simulink model "ieee30"  (R2017a)
settings: Solver=VariableStepDiscrete  StartTime=0.0  StopTime=0.012  MaxStep=1e-4  RelTol=1e-3
undefined symbols (not defined in the file): Angle, Magnitude
libraries: powerlib x548
(part 3 of 4)

== system ieee30/Bus29 ==
  I2927 : powerlib/Measurements/Three-Phase V-I Measurement  VoltageMeasurement=no  SetLabelV=off  LabelV=Vabc  Vpu=off  VpuLL=off  CurrentMeasurement=yes  SetLabelI=on  LabelI=I2927  Ipu=off  Pbase=100e6  Vbase=500e3  OutputType=Magnitude-Angle  PhasorSimulation=on  PSBequivalent=0
  Load29 : powerlib/Measurements/Three-Phase V-I Measurement  VoltageMeasurement=no  SetLabelV=off  LabelV=V21  Vpu=off  VpuLL=off  CurrentMeasurement=no  SetLabelI=off  LabelI=I2224  Ipu=off  Pbase=100e6  Vbase=500e3  OutputType=Complex  PhasorSimulation=on  PSBequivalent=0
  To Workspace1 : ToWorkspace  VariableName=V29  SaveFormat=Timeseries  SampleTime=0.01
  To Workspace2 : ToWorkspace  VariableName=I2927  SaveFormat=Timeseries  SampleTime=0.01
  To Workspace3 : ToWorkspace  VariableName=I2930  SaveFormat=Timeseries  SampleTime=0.01
  V29 I2930 : powerlib/Measurements/Three-Phase V-I Measurement  VoltageMeasurement=phase-to-phase  SetLabelV=on  LabelV=V29  Vpu=off  VpuLL=off  CurrentMeasurement=yes  SetLabelI=on  LabelI=I2930  Ipu=off  Pbase=100e6  Vbase=500e3  OutputType=Magnitude-Angle  PhasorSimulation=on  PSBequivalent=0
  I2930A : PMIOPort  Port=1  Side=Right
  I2930B : PMIOPort  Port=2  Side=Right
  I2930C : PMIOPort  Port=3  Side=Right
  I2927A : PMIOPort  Port=4  Side=Right
  I2927B : PMIOPort  Port=5  Side=Right
  I2927C : PMIOPort  Port=6  Side=Right
  Load29A : PMIOPort  Port=7  Side=Left
  Load29B : PMIOPort  Port=8  Side=Left
  Load29C : PMIOPort  Port=9  Side=Left
  wires:
  [V29] -> To Workspace1/1
  [I2927] -> To Workspace2/1
  [I2930] -> To Workspace3/1
  connections:
  V29 I2930/RConn2 -- I2930B/RConn1
  I2927/RConn1 -- I2927A/RConn1
  V29 I2930/RConn1 -- I2930A/RConn1
  I2927/RConn2 -- I2927B/RConn1
  I2927/RConn3 -- I2927C/RConn1
  V29 I2930/RConn3 -- I2930C/RConn1
  V29 I2930/LConn1 -- Load29/LConn1 -- I2927/LConn1
  V29 I2930/LConn2 -- Load29/LConn2 -- I2927/LConn2
  V29 I2930/LConn3 -- Load29/LConn3 -- I2927/LConn3
  Load29/RConn1 -- Load29A/RConn1
  Load29/RConn2 -- Load29B/RConn1
  Load29/RConn3 -- Load29C/RConn1

== system ieee30/Bus3 ==
  I34 : powerlib/Measurements/Three-Phase V-I Measurement  VoltageMeasurement=no  SetLabelV=off  LabelV=V3  Vpu=off  VpuLL=off  CurrentMeasurement=yes  SetLabelI=on  LabelI=I34  Ipu=off  Pbase=100e6  Vbase=500e3  OutputType=Magnitude-Angle  PhasorSimulation=on  PSBequivalent=0
  Load3 : powerlib/Measurements/Three-Phase V-I Measurement  VoltageMeasurement=no  SetLabelV=off  LabelV=V3  Vpu=off  VpuLL=off  CurrentMeasurement=no  SetLabelI=off  LabelI=I31  Ipu=off  Pbase=100e6  Vbase=500e3  OutputType=Complex  PhasorSimulation=on  PSBequivalent=0
  To Workspace1 : ToWorkspace  VariableName=I34  SaveFormat=Timeseries  SampleTime=0.01
  To Workspace2 : ToWorkspace  VariableName=I31  SaveFormat=Timeseries  SampleTime=0.01
  To Workspace3 : ToWorkspace  VariableName=V3  SaveFormat=Timeseries  SampleTime=0.01
  V3 I31 : powerlib/Measurements/Three-Phase V-I Measurement  VoltageMeasurement=phase-to-phase  SetLabelV=on  LabelV=V3  Vpu=off  VpuLL=off  CurrentMeasurement=yes  SetLabelI=on  LabelI=I31  Ipu=off  Pbase=100e6  Vbase=500e3  OutputType=Magnitude-Angle  PhasorSimulation=on  PSBequivalent=0
  I31A : PMIOPort  Port=1  Side=Left
  I31B : PMIOPort  Port=2  Side=Left
  I31C : PMIOPort  Port=3  Side=Left
  Load3A : PMIOPort  Port=4  Side=Left
  Load3B : PMIOPort  Port=5  Side=Left
  Load3C : PMIOPort  Port=6  Side=Left
  I34A : PMIOPort  Port=7  Side=Right
  I34B : PMIOPort  Port=8  Side=Right
  I34C : PMIOPort  Port=9  Side=Right
  wires:
  [I31] -> To Workspace2/1
  [V3] -> To Workspace3/1
  [I34] -> To Workspace1/1
  connections:
  I31A/RConn1 -- V3 I31/RConn1
  I31B/RConn1 -- V3 I31/RConn2
  I31C/RConn1 -- V3 I31/RConn3
  Load3/RConn3 -- Load3C/RConn1
  Load3/RConn1 -- Load3A/RConn1
  Load3/RConn2 -- Load3B/RConn1
  I34/RConn3 -- I34C/RConn1
  I34/RConn1 -- I34A/RConn1
  I34/RConn2 -- I34B/RConn1
  V3 I31/LConn1 -- I34/LConn1 -- Load3/LConn1
  V3 I31/LConn2 -- Load3/LConn2 -- I34/LConn2
  V3 I31/LConn3 -- Load3/LConn3 -- I34/LConn3

== system ieee30/Bus30 ==
  I3029 : powerlib/Measurements/Three-Phase V-I Measurement  VoltageMeasurement=no  SetLabelV=off  LabelV=Vabc  Vpu=off  VpuLL=off  CurrentMeasurement=yes  SetLabelI=on  LabelI=I3029  Ipu=off  Pbase=100e6  Vbase=500e3  OutputType=Magnitude-Angle  PhasorSimulation=on  PSBequivalent=0
  Load30 : powerlib/Measurements/Three-Phase V-I Measurement  VoltageMeasurement=no  SetLabelV=off  LabelV=V21  Vpu=off  VpuLL=off  CurrentMeasurement=no  SetLabelI=off  LabelI=I2224  Ipu=off  Pbase=100e6  Vbase=500e3  OutputType=Complex  PhasorSimulation=on  PSBequivalent=0
  To Workspace1 : ToWorkspace  VariableName=V30  SaveFormat=Timeseries  SampleTime=0.01
  To Workspace2 : ToWorkspace  VariableName=I3027  SaveFormat=Timeseries  SampleTime=0.01
  To Workspace3 : ToWorkspace  VariableName=I3029  SaveFormat=Timeseries  SampleTime=0.01
  V30 I3027 : powerlib/Measurements/Three-Phase V-I Measurement  VoltageMeasurement=phase-to-phase  SetLabelV=on  LabelV=V30  Vpu=off  VpuLL=off  CurrentMeasurement=yes  SetLabelI=on  LabelI=I3027  Ipu=off  Pbase=100e6  Vbase=500e3  OutputType=Magnitude-Angle  PhasorSimulation=on  PSBequivalent=0
  I3029A : PMIOPort  Port=1  Side=Right
  I3029B : PMIOPort  Port=2  Side=Right
  I3029C : PMIOPort  Port=3  Side=Right
  I3027A : PMIOPort  Port=4  Side=Right
  I3027B : PMIOPort  Port=5  Side=Right
  I3027C : PMIOPort  Port=6  Side=Right
  Load30A : PMIOPort  Port=7  Side=Left
  Load30B : PMIOPort  Port=8  Side=Left
  Load30C : PMIOPort  Port=9  Side=Left
  wires:
  [V30] -> To Workspace1/1
  [I3027] -> To Workspace2/1
  [I3029] -> To Workspace3/1
  connections:
  V30 I3027/RConn2 -- I3027B/RConn1
  I3029/RConn1 -- I3029A/RConn1
  V30 I3027/RConn1 -- I3027A/RConn1
  I3029/RConn2 -- I3029B/RConn1
  I3029/RConn3 -- I3029C/RConn1
  V30 I3027/RConn3 -- I3027C/RConn1
  V30 I3027/LConn1 -- Load30/LConn1 -- I3029/LConn1
  V30 I3027/LConn2 -- Load30/LConn2 -- I3029/LConn2
  V30 I3027/LConn3 -- Load30/LConn3 -- I3029/LConn3
  Load30/RConn1 -- Load30A/RConn1
  Load30/RConn2 -- Load30B/RConn1
  Load30/RConn3 -- Load30C/RConn1

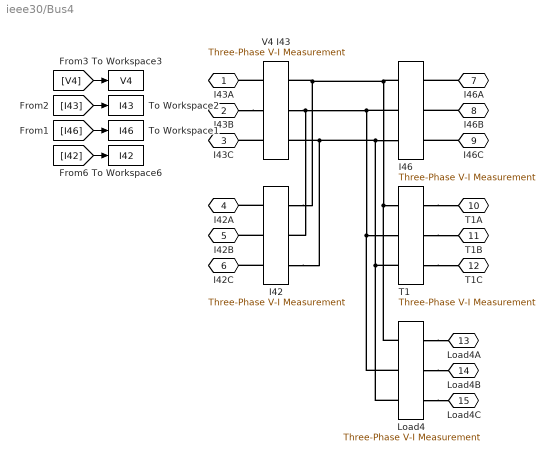
== system ieee30/Bus4 ==
  I42 : powerlib/Measurements/Three-Phase V-I Measurement  VoltageMeasurement=no  SetLabelV=off  LabelV=V4  Vpu=off  VpuLL=off  CurrentMeasurement=yes  SetLabelI=on  LabelI=I42  Ipu=off  Pbase=100e6  Vbase=500e3  OutputType=Magnitude-Angle  PhasorSimulation=on  PSBequivalent=0
  I46 : powerlib/Measurements/Three-Phase V-I Measurement  VoltageMeasurement=no  SetLabelV=off  LabelV=V4  Vpu=off  VpuLL=off  CurrentMeasurement=yes  SetLabelI=on  LabelI=I46  Ipu=off  Pbase=100e6  Vbase=500e3  OutputType=Magnitude-Angle  PhasorSimulation=on  PSBequivalent=0
  Load4 : powerlib/Measurements/Three-Phase V-I Measurement  VoltageMeasurement=no  SetLabelV=off  LabelV=V4  Vpu=off  VpuLL=off  CurrentMeasurement=no  SetLabelI=off  LabelI=I412  Ipu=off  Pbase=100e6  Vbase=500e3  OutputType=Complex  PhasorSimulation=on  PSBequivalent=0
  T1 : powerlib/Measurements/Three-Phase V-I Measurement  VoltageMeasurement=no  SetLabelV=off  LabelV=V4  Vpu=off  VpuLL=off  CurrentMeasurement=no  SetLabelI=off  LabelI=I412  Ipu=off  Pbase=100e6  Vbase=500e3  OutputType=Complex  PhasorSimulation=on  PSBequivalent=0
  To Workspace1 : ToWorkspace  VariableName=I46  SaveFormat=Timeseries  SampleTime=0.01
  To Workspace2 : ToWorkspace  VariableName=I43  SaveFormat=Timeseries  SampleTime=0.01
  To Workspace3 : ToWorkspace  VariableName=V4  SaveFormat=Timeseries  SampleTime=0.01
  To Workspace6 : ToWorkspace  VariableName=I42  SaveFormat=Timeseries  SampleTime=0.01
  V4 I43 : powerlib/Measurements/Three-Phase V-I Measurement  VoltageMeasurement=phase-to-phase  SetLabelV=on  LabelV=V4  Vpu=off  VpuLL=off  CurrentMeasurement=yes  SetLabelI=on  LabelI=I43  Ipu=off  Pbase=100e6  Vbase=500e3  OutputType=Magnitude-Angle  PhasorSimulation=on  PSBequivalent=0
  I43A : PMIOPort  Port=1  Side=Left
  I43B : PMIOPort  Port=2  Side=Left
  I43C : PMIOPort  Port=3  Side=Left
  I42A : PMIOPort  Port=4  Side=Left
  I42B : PMIOPort  Port=5  Side=Left
  I42C : PMIOPort  Port=6  Side=Left
  I46A : PMIOPort  Port=7  Side=Left
  I46B : PMIOPort  Port=8  Side=Left
  I46C : PMIOPort  Port=9  Side=Left
  T1A : PMIOPort  Port=10  Side=Right
  T1B : PMIOPort  Port=11  Side=Right
  T1C : PMIOPort  Port=12  Side=Right
  Load4A : PMIOPort  Port=13  Side=Right
  Load4B : PMIOPort  Port=14  Side=Right
  Load4C : PMIOPort  Port=15  Side=Right
  wires:
  [I46] -> To Workspace1/1
  [V4] -> To Workspace3/1
  [I43] -> To Workspace2/1
  [I42] -> To Workspace6/1
  connections:
  I43B/RConn1 -- V4 I43/RConn2
  V4 I43/RConn1 -- I43A/RConn1
  V4 I43/RConn3 -- I43C/RConn1
  T1/LConn3 -- V4 I43/LConn3 -- I42/LConn3 -- I46/LConn3 -- Load4/LConn3
  I46/LConn1 -- Load4/LConn1 -- T1/LConn1 -- I42/LConn1 -- V4 I43/LConn1
  V4 I43/LConn2 -- I46/LConn2 -- Load4/LConn2 -- T1/LConn2 -- I42/LConn2
  I42/RConn1 -- I42A/RConn1
  I42/RConn2 -- I42B/RConn1
  I42/RConn3 -- I42C/RConn1
  I46A/RConn1 -- I46/RConn1
  I46B/RConn1 -- I46/RConn2
  I46C/RConn1 -- I46/RConn3
  T1/RConn1 -- T1A/RConn1
  T1/RConn3 -- T1C/RConn1
  T1/RConn2 -- T1B/RConn1
  Load4/RConn1 -- Load4A/RConn1
  Load4/RConn2 -- Load4B/RConn1
  Load4/RConn3 -- Load4C/RConn1

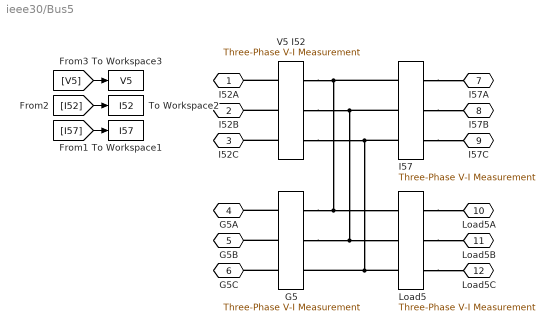
== system ieee30/Bus5 ==
  G5 : powerlib/Measurements/Three-Phase V-I Measurement  VoltageMeasurement=no  SetLabelV=off  LabelV=V5  Vpu=off  VpuLL=off  CurrentMeasurement=no  SetLabelI=off  LabelI=I52  Ipu=off  Pbase=100e6  Vbase=500e3  OutputType=Complex  PhasorSimulation=on  PSBequivalent=0
  I57 : powerlib/Measurements/Three-Phase V-I Measurement  VoltageMeasurement=no  SetLabelV=off  LabelV=V5  Vpu=off  VpuLL=off  CurrentMeasurement=yes  SetLabelI=on  LabelI=I57  Ipu=off  Pbase=100e6  Vbase=500e3  OutputType=Magnitude-Angle  PhasorSimulation=on  PSBequivalent=0
  Load5 : powerlib/Measurements/Three-Phase V-I Measurement  VoltageMeasurement=no  SetLabelV=off  LabelV=V5  Vpu=off  VpuLL=off  CurrentMeasurement=no  SetLabelI=off  LabelI=I52  Ipu=off  Pbase=100e6  Vbase=500e3  OutputType=Complex  PhasorSimulation=on  PSBequivalent=0
  To Workspace1 : ToWorkspace  VariableName=I57  SaveFormat=Timeseries  SampleTime=0.01
  To Workspace2 : ToWorkspace  VariableName=I52  SaveFormat=Timeseries  SampleTime=0.01
  To Workspace3 : ToWorkspace  VariableName=V5  SaveFormat=Timeseries  SampleTime=0.01
  V5 I52 : powerlib/Measurements/Three-Phase V-I Measurement  VoltageMeasurement=phase-to-phase  SetLabelV=on  LabelV=V5  Vpu=off  VpuLL=off  CurrentMeasurement=yes  SetLabelI=on  LabelI=I52  Ipu=off  Pbase=100e6  Vbase=500e3  OutputType=Magnitude-Angle  PhasorSimulation=on  PSBequivalent=0
  I52A : PMIOPort  Port=1  Side=Left
  I52B : PMIOPort  Port=2  Side=Left
  I52C : PMIOPort  Port=3  Side=Left
  G5A : PMIOPort  Port=4  Side=Right
  G5B : PMIOPort  Port=5  Side=Right
  G5C : PMIOPort  Port=6  Side=Right
  I57A : PMIOPort  Port=7  Side=Left
  I57B : PMIOPort  Port=8  Side=Left
  I57C : PMIOPort  Port=9  Side=Left
  Load5A : PMIOPort  Port=10  Side=Right
  Load5B : PMIOPort  Port=11  Side=Right
  Load5C : PMIOPort  Port=12  Side=Right
  wires:
  [I57] -> To Workspace1/1
  [V5] -> To Workspace3/1
  [I52] -> To Workspace2/1
  connections:
  V5 I52/RConn3 -- I52C/RConn1
  V5 I52/RConn2 -- I52B/RConn1
  V5 I52/RConn1 -- I52A/RConn1
  V5 I52/LConn1 -- I57/LConn1 -- Load5/LConn1 -- G5/LConn1
  V5 I52/LConn2 -- I57/LConn2 -- Load5/LConn2 -- G5/LConn2
  V5 I52/LConn3 -- I57/LConn3 -- G5/LConn3 -- Load5/LConn3
  G5/RConn1 -- G5A/RConn1
  G5/RConn3 -- G5C/RConn1
  G5/RConn2 -- G5B/RConn1
  I57/RConn3 -- I57C/RConn1
  I57/RConn1 -- I57A/RConn1
  I57/RConn2 -- I57B/RConn1
  Load5/RConn1 -- Load5A/RConn1
  Load5/RConn2 -- Load5B/RConn1
  Load5/RConn3 -- Load5C/RConn1

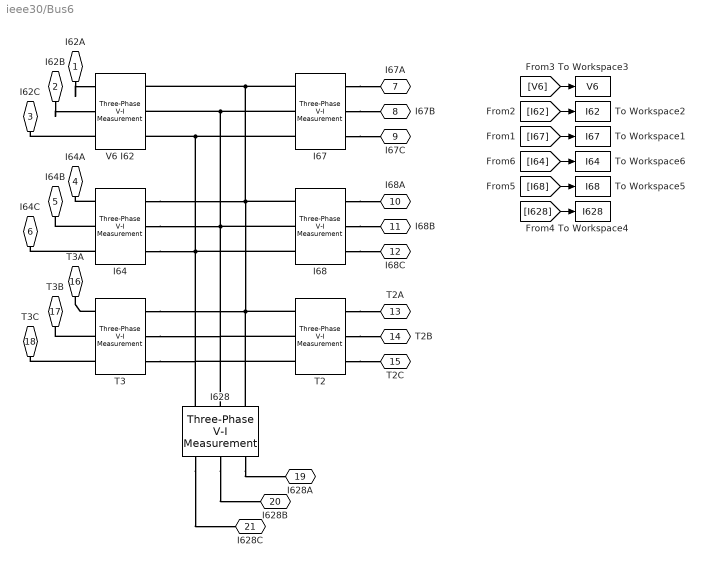
== system ieee30/Bus6 ==
  I628 : powerlib/Measurements/Three-Phase V-I Measurement  VoltageMeasurement=no  SetLabelV=off  LabelV=Vabc  Vpu=off  VpuLL=off  CurrentMeasurement=yes  SetLabelI=on  LabelI=I628  Ipu=off  Pbase=100e6  Vbase=500e3  OutputType=Magnitude-Angle  PhasorSimulation=on  PSBequivalent=0
  I64 : powerlib/Measurements/Three-Phase V-I Measurement  VoltageMeasurement=no  SetLabelV=off  LabelV=V6  Vpu=off  VpuLL=off  CurrentMeasurement=yes  SetLabelI=on  LabelI=I64  Ipu=off  Pbase=100e6  Vbase=500e3  OutputType=Magnitude-Angle  PhasorSimulation=on  PSBequivalent=0
  I67 : powerlib/Measurements/Three-Phase V-I Measurement  VoltageMeasurement=no  SetLabelV=off  LabelV=Vabc  Vpu=off  VpuLL=off  CurrentMeasurement=yes  SetLabelI=on  LabelI=I67  Ipu=off  Pbase=100e6  Vbase=500e3  OutputType=Magnitude-Angle  PhasorSimulation=on  PSBequivalent=0
  I68 : powerlib/Measurements/Three-Phase V-I Measurement  VoltageMeasurement=no  SetLabelV=off  LabelV=Vabc  Vpu=off  VpuLL=off  CurrentMeasurement=yes  SetLabelI=on  LabelI=I68  Ipu=off  Pbase=100e6  Vbase=500e3  OutputType=Magnitude-Angle  PhasorSimulation=on  PSBequivalent=0
  T2 : powerlib/Measurements/Three-Phase V-I Measurement  VoltageMeasurement=no  SetLabelV=off  LabelV=Vabc  Vpu=off  VpuLL=off  CurrentMeasurement=no  SetLabelI=off  LabelI=I69  Ipu=off  Pbase=100e6  Vbase=500e3  OutputType=Complex  PhasorSimulation=on  PSBequivalent=0
  T3 : powerlib/Measurements/Three-Phase V-I Measurement  VoltageMeasurement=no  SetLabelV=off  LabelV=Vabc  Vpu=off  VpuLL=off  CurrentMeasurement=no  SetLabelI=off  LabelI=I69  Ipu=off  Pbase=100e6  Vbase=500e3  OutputType=Complex  PhasorSimulation=on  PSBequivalent=0
  To Workspace1 : ToWorkspace  VariableName=I67  SaveFormat=Timeseries  SampleTime=0.01
  To Workspace2 : ToWorkspace  VariableName=I62  SaveFormat=Timeseries  SampleTime=0.01
  To Workspace3 : ToWorkspace  VariableName=V6  SaveFormat=Timeseries  SampleTime=0.01
  To Workspace4 : ToWorkspace  VariableName=I628  SaveFormat=Timeseries  SampleTime=0.01
  To Workspace5 : ToWorkspace  VariableName=I68  SaveFormat=Timeseries  SampleTime=0.01
  To Workspace6 : ToWorkspace  VariableName=I64  SaveFormat=Timeseries  SampleTime=0.01
  V6 I62 : powerlib/Measurements/Three-Phase V-I Measurement  VoltageMeasurement=phase-to-phase  SetLabelV=on  LabelV=V6  Vpu=off  VpuLL=off  CurrentMeasurement=yes  SetLabelI=on  LabelI=I62  Ipu=off  Pbase=100e6  Vbase=500e3  OutputType=Magnitude-Angle  PhasorSimulation=on  PSBequivalent=0
  I62A : PMIOPort  Port=1  Side=Left
  I62B : PMIOPort  Port=2  Side=Left
  I62C : PMIOPort  Port=3  Side=Left
  I64A : PMIOPort  Port=4  Side=Right
  I64B : PMIOPort  Port=5  Side=Right
  I64C : PMIOPort  Port=6  Side=Right
  I67A : PMIOPort  Port=7  Side=Left
  I67B : PMIOPort  Port=8  Side=Left
  I67C : PMIOPort  Port=9  Side=Left
  I68A : PMIOPort  Port=10  Side=Left
  I68B : PMIOPort  Port=11  Side=Left
  I68C : PMIOPort  Port=12  Side=Left
  T2A : PMIOPort  Port=13  Side=Right
  T2B : PMIOPort  Port=14  Side=Right
  T2C : PMIOPort  Port=15  Side=Right
  T3A : PMIOPort  Port=16  Side=Right
  T3B : PMIOPort  Port=17  Side=Right
  T3C : PMIOPort  Port=18  Side=Right
  I628A : PMIOPort  Port=19  Side=Right
  I628B : PMIOPort  Port=20  Side=Right
  I628C : PMIOPort  Port=21  Side=Right
  wires:
  [I67] -> To Workspace1/1
  [V6] -> To Workspace3/1
  [I62] -> To Workspace2/1
  [I628] -> To Workspace4/1
  [I64] -> To Workspace6/1
  [I68] -> To Workspace5/1
  connections:
  I62A/RConn1 -- V6 I62/RConn1
  I62B/RConn1 -- V6 I62/RConn2
  I64/LConn1 -- I68/LConn1 -- I67/LConn1 -- V6 I62/LConn1 -- I628/LConn3 -- T3/LConn1 -- T2/LConn1
  I64/LConn2 -- I68/LConn2 -- I67/LConn2 -- V6 I62/LConn2 -- I628/LConn2 -- T3/LConn2 -- T2/LConn2
  I64/LConn3 -- I68/LConn3 -- I67/LConn3 -- V6 I62/LConn3 -- I628/LConn1 -- T3/LConn3 -- T2/LConn3
  V6 I62/RConn3 -- I62C/RConn1
  I64/RConn3 -- I64C/RConn1
  I64/RConn2 -- I64B/RConn1
  I64/RConn1 -- I64A/RConn1
  I67/RConn1 -- I67A/RConn1
  I67/RConn3 -- I67C/RConn1
  I67/RConn2 -- I67B/RConn1
  I68/RConn3 -- I68C/RConn1
  I68/RConn1 -- I68A/RConn1
  I68/RConn2 -- I68B/RConn1
  T2/RConn2 -- T2B/RConn1
  T2/RConn3 -- T2C/RConn1
  T2/RConn1 -- T2A/RConn1
  T3/RConn3 -- T3C/RConn1
  T3/RConn1 -- T3A/RConn1
  T3/RConn2 -- T3B/RConn1
  I628/RConn1 -- I628C/RConn1
  I628/RConn3 -- I628A/RConn1
  I628/RConn2 -- I628B/RConn1

== system ieee30/Bus7 ==
  I76 : powerlib/Measurements/Three-Phase V-I Measurement  VoltageMeasurement=no  SetLabelV=off  LabelV=V7  Vpu=off  VpuLL=off  CurrentMeasurement=yes  SetLabelI=on  LabelI=I76  Ipu=off  Pbase=100e6  Vbase=500e3  OutputType=Magnitude-Angle  PhasorSimulation=on  PSBequivalent=0
  Load7 : powerlib/Measurements/Three-Phase V-I Measurement  VoltageMeasurement=no  SetLabelV=off  LabelV=V7  Vpu=off  VpuLL=off  CurrentMeasurement=no  SetLabelI=off  LabelI=I57  Ipu=off  Pbase=100e6  Vbase=500e3  OutputType=Complex  PhasorSimulation=on  PSBequivalent=0
  To Workspace1 : ToWorkspace  VariableName=I76  SaveFormat=Timeseries  SampleTime=0.01
  To Workspace2 : ToWorkspace  VariableName=I75  SaveFormat=Timeseries  SampleTime=0.01
  To Workspace3 : ToWorkspace  VariableName=V7  SaveFormat=Timeseries  SampleTime=0.01
  V7 I75 : powerlib/Measurements/Three-Phase V-I Measurement  VoltageMeasurement=phase-to-phase  SetLabelV=on  LabelV=V7  Vpu=off  VpuLL=off  CurrentMeasurement=yes  SetLabelI=on  LabelI=I75  Ipu=off  Pbase=100e6  Vbase=500e3  OutputType=Magnitude-Angle  PhasorSimulation=on  PSBequivalent=0
  Load7A : PMIOPort  Port=1  Side=Left
  Load7B : PMIOPort  Port=2  Side=Left
  Load7C : PMIOPort  Port=3  Side=Left
  I75A : PMIOPort  Port=4  Side=Left
  I75B : PMIOPort  Port=5  Side=Left
  I75C : PMIOPort  Port=6  Side=Left
  I76A : PMIOPort  Port=7  Side=Left
  I76B : PMIOPort  Port=8  Side=Left
  I76C : PMIOPort  Port=9  Side=Left
  wires:
  [I76] -> To Workspace1/1
  [V7] -> To Workspace3/1
  [I75] -> To Workspace2/1
  connections:
  I76/RConn3 -- I76C/RConn1
  V7 I75/RConn3 -- I75C/RConn1
  V7 I75/RConn2 -- I75B/RConn1
  V7 I75/RConn1 -- I75A/RConn1
  I76/RConn2 -- I76B/RConn1
  I76/RConn1 -- I76A/RConn1
  V7 I75/LConn1 -- Load7/LConn1 -- I76/LConn1
  V7 I75/LConn2 -- Load7/LConn2 -- I76/LConn2
  I76/LConn3 -- Load7/LConn3 -- V7 I75/LConn3
  Load7A/RConn1 -- Load7/RConn1
  Load7/RConn2 -- Load7B/RConn1
  Load7C/RConn1 -- Load7/RConn3

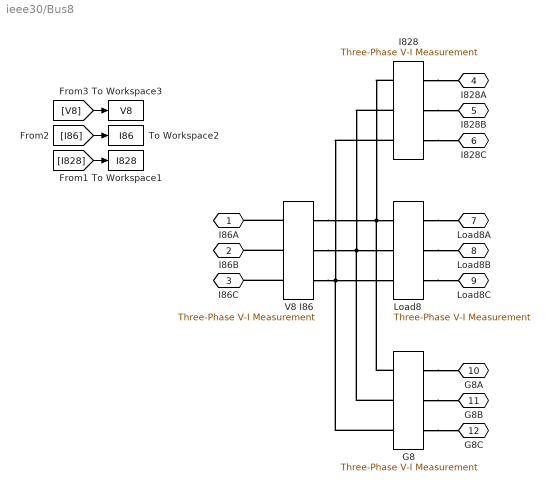
== system ieee30/Bus8 ==
  G8 : powerlib/Measurements/Three-Phase V-I Measurement  VoltageMeasurement=no  SetLabelV=off  LabelV=Vabc  Vpu=off  VpuLL=off  CurrentMeasurement=no  SetLabelI=off  LabelI=Iabc  Ipu=off  Pbase=100e6  Vbase=500e3  OutputType=Complex  PhasorSimulation=on  PSBequivalent=0
  I828 : powerlib/Measurements/Three-Phase V-I Measurement  VoltageMeasurement=no  SetLabelV=off  LabelV=V8  Vpu=off  VpuLL=off  CurrentMeasurement=yes  SetLabelI=on  LabelI=I828  Ipu=off  Pbase=100e6  Vbase=500e3  OutputType=Magnitude-Angle  PhasorSimulation=on  PSBequivalent=0
  Load8 : powerlib/Measurements/Three-Phase V-I Measurement  VoltageMeasurement=no  SetLabelV=off  LabelV=Vabc  Vpu=off  VpuLL=off  CurrentMeasurement=no  SetLabelI=off  LabelI=Iabc  Ipu=off  Pbase=100e6  Vbase=500e3  OutputType=Complex  PhasorSimulation=on  PSBequivalent=0
  To Workspace1 : ToWorkspace  VariableName=I828  SaveFormat=Timeseries  SampleTime=0.01
  To Workspace2 : ToWorkspace  VariableName=I86  SaveFormat=Timeseries  SampleTime=0.01
  To Workspace3 : ToWorkspace  VariableName=V8  SaveFormat=Timeseries  SampleTime=0.01
  V8 I86 : powerlib/Measurements/Three-Phase V-I Measurement  VoltageMeasurement=phase-to-phase  SetLabelV=on  LabelV=V8  Vpu=off  VpuLL=off  CurrentMeasurement=yes  SetLabelI=on  LabelI=I86  Ipu=off  Pbase=100e6  Vbase=500e3  OutputType=Magnitude-Angle  PhasorSimulation=on  PSBequivalent=0
  I86A : PMIOPort  Port=1  Side=Left
  I86B : PMIOPort  Port=2  Side=Left
  I86C : PMIOPort  Port=3  Side=Left
  I828A : PMIOPort  Port=4  Side=Right
  I828B : PMIOPort  Port=5  Side=Right
  I828C : PMIOPort  Port=6  Side=Right
  Load8A : PMIOPort  Port=7  Side=Right
  Load8B : PMIOPort  Port=8  Side=Right
  Load8C : PMIOPort  Port=9  Side=Right
  G8A : PMIOPort  Port=10  Side=Right
  G8B : PMIOPort  Port=11  Side=Right
  G8C : PMIOPort  Port=12  Side=Right
  wires:
  [I828] -> To Workspace1/1
  [V8] -> To Workspace3/1
  [I86] -> To Workspace2/1
  connections:
  V8 I86/RConn3 -- I86C/RConn1
  Load8/RConn3 -- Load8C/RConn1
  Load8/RConn2 -- Load8B/RConn1
  V8 I86/RConn2 -- I86B/RConn1
  Load8/RConn1 -- Load8A/RConn1
  V8 I86/RConn1 -- I86A/RConn1
  V8 I86/LConn1 -- I828/LConn1 -- G8/LConn1 -- Load8/LConn1
  V8 I86/LConn2 -- I828/LConn2 -- G8/LConn2 -- Load8/LConn2
  V8 I86/LConn3 -- I828/LConn3 -- G8/LConn3 -- Load8/LConn3
  G8/RConn2 -- G8B/RConn1
  G8/RConn1 -- G8A/RConn1
  G8/RConn3 -- G8C/RConn1
  I828/RConn3 -- I828C/RConn1
  I828/RConn2 -- I828B/RConn1
  I828/RConn1 -- I828A/RConn1

== system ieee30/Bus9 ==
  T3 : powerlib/Measurements/Three-Phase V-I Measurement  VoltageMeasurement=no  SetLabelV=off  LabelV=Vabc  Vpu=off  VpuLL=off  CurrentMeasurement=no  SetLabelI=off  LabelI=Iabc  Ipu=off  Pbase=100e6  Vbase=500e3  OutputType=Complex  PhasorSimulation=on  PSBequivalent=0
  T3_910 : powerlib/Measurements/Three-Phase V-I Measurement  VoltageMeasurement=no  SetLabelV=off  LabelV=Vabc  Vpu=off  VpuLL=off  CurrentMeasurement=no  SetLabelI=off  LabelI=Iabc  Ipu=off  Pbase=100e6  Vbase=500e3  OutputType=Complex  PhasorSimulation=on  PSBequivalent=0
  T3_911 : powerlib/Measurements/Three-Phase V-I Measurement  VoltageMeasurement=no  SetLabelV=off  LabelV=Vabc  Vpu=off  VpuLL=off  CurrentMeasurement=no  SetLabelI=off  LabelI=Iabc  Ipu=off  Pbase=100e6  Vbase=500e3  OutputType=Complex  PhasorSimulation=on  PSBequivalent=0
  T3A : PMIOPort  Port=1  Side=Left
  T3B : PMIOPort  Port=2  Side=Left
  T3C : PMIOPort  Port=3  Side=Left
  T3_910A : PMIOPort  Port=4  Side=Right
  T3_910B : PMIOPort  Port=5  Side=Right
  T3_910C : PMIOPort  Port=6  Side=Right
  T3_911A : PMIOPort  Port=7  Side=Right
  T3_911B : PMIOPort  Port=8  Side=Right
  T3_911C : PMIOPort  Port=9  Side=Right
  connections:
  T3/RConn1 -- T3A/RConn1
  T3/RConn2 -- T3B/RConn1
  T3/RConn3 -- T3C/RConn1
  T3_910/LConn1 -- T3_911/LConn1 -- T3/LConn1
  T3_910/LConn2 -- T3_911/LConn2 -- T3/LConn2
  T3_910/LConn3 -- T3_911/LConn3 -- T3/LConn3
  T3_910A/RConn1 -- T3_910/RConn1
  T3_910B/RConn1 -- T3_910/RConn2
  T3_910C/RConn1 -- T3_910/RConn3
  T3_911/RConn3 -- T3_911C/RConn1
  T3_911/RConn1 -- T3_911A/RConn1
  T3_911/RConn2 -- T3_911B/RConn1

== system ieee30/Line 1-2-1 ==
  Line{,1..4} (5 alike) : powerlib/Elements/Three-Phase PI Section Line  LConnTagsString=a|b|c  RConnTagsString=A|B|C  Frequency=60  Resistances=[rt ro] /100  Inductances=[ lt lo] /100  Capacitances=[ct co]/100  Length=20
      settings: SourceProductName=Simscape Power Systems
  A : PMIOPort  Port=1  Side=Left
  B : PMIOPort  Port=2  Side=Left
  C : PMIOPort  Port=3  Side=Left
  a : PMIOPort  Port=4  Side=Right
  b : PMIOPort  Port=5  Side=Right
  c : PMIOPort  Port=6  Side=Right
  connections:
  Line3/RConn3 -- Line4/LConn3
  Line/RConn3 -- Line1/LConn3
  Line2/RConn3 -- Line3/LConn3
  Line2/RConn1 -- Line3/LConn1
  Line1/RConn3 -- Line2/LConn3
  Line/RConn2 -- Line1/LConn2
  Line2/RConn2 -- Line3/LConn2
  Line1/RConn1 -- Line2/LConn1
  Line3/RConn1 -- Line4/LConn1
  Line3/RConn2 -- Line4/LConn2
  Line1/RConn2 -- Line2/LConn2
  Line/RConn1 -- Line1/LConn1
  C/RConn1 -- Line/LConn3
  Line/LConn1 -- A/RConn1
  c/RConn1 -- Line4/RConn3
  a/RConn1 -- Line4/RConn1
  B/RConn1 -- Line/LConn2
  b/RConn1 -- Line4/RConn2

== system ieee30/Line 1-2-2 ==
  Line{,1..4} (5 alike) : powerlib/Elements/Three-Phase PI Section Line  LConnTagsString=a|b|c  RConnTagsString=A|B|C  Frequency=60  Resistances=[rt ro] /100  Inductances=[ lt lo] /100  Capacitances=[ct co]/100  Length=20
      settings: SourceProductName=Simscape Power Systems
  A : PMIOPort  Port=1  Side=Left
  B : PMIOPort  Port=2  Side=Left
  C : PMIOPort  Port=3  Side=Left
  a : PMIOPort  Port=4  Side=Right
  b : PMIOPort  Port=5  Side=Right
  c : PMIOPort  Port=6  Side=Right
  connections:
  Line3/RConn3 -- Line4/LConn3
  Line/RConn3 -- Line1/LConn3
  Line2/RConn3 -- Line3/LConn3
  Line2/RConn1 -- Line3/LConn1
  Line1/RConn3 -- Line2/LConn3
  Line/RConn2 -- Line1/LConn2
  Line2/RConn2 -- Line3/LConn2
  Line1/RConn1 -- Line2/LConn1
  Line3/RConn1 -- Line4/LConn1
  Line3/RConn2 -- Line4/LConn2
  Line1/RConn2 -- Line2/LConn2
  Line/RConn1 -- Line1/LConn1
  C/RConn1 -- Line/LConn3
  Line/LConn1 -- A/RConn1
  c/RConn1 -- Line4/RConn3
  a/RConn1 -- Line4/RConn1
  B/RConn1 -- Line/LConn2
  b/RConn1 -- Line4/RConn2

== system ieee30/Line 1-3-1 ==
  Line{,1..4} (5 alike) : powerlib/Elements/Three-Phase PI Section Line  LConnTagsString=a|b|c  RConnTagsString=A|B|C  Frequency=60  Resistances=[rt ro] /100  Inductances=[ lt lo] /100  Capacitances=[ct co]/100  Length=20
      settings: SourceProductName=Simscape Power Systems
  A : PMIOPort  Port=1  Side=Left
  B : PMIOPort  Port=2  Side=Left
  C : PMIOPort  Port=3  Side=Left
  a : PMIOPort  Port=4  Side=Right
  b : PMIOPort  Port=5  Side=Right
  c : PMIOPort  Port=6  Side=Right
  connections:
  Line3/RConn3 -- Line4/LConn3
  Line/RConn3 -- Line1/LConn3
  Line2/RConn3 -- Line3/LConn3
  Line2/RConn1 -- Line3/LConn1
  Line1/RConn3 -- Line2/LConn3
  Line/RConn2 -- Line1/LConn2
  Line2/RConn2 -- Line3/LConn2
  Line1/RConn1 -- Line2/LConn1
  Line3/RConn1 -- Line4/LConn1
  Line3/RConn2 -- Line4/LConn2
  Line1/RConn2 -- Line2/LConn2
  Line/RConn1 -- Line1/LConn1
  C/RConn1 -- Line/LConn3
  Line/LConn1 -- A/RConn1
  c/RConn1 -- Line4/RConn3
  a/RConn1 -- Line4/RConn1
  B/RConn1 -- Line/LConn2
  b/RConn1 -- Line4/RConn2

== system ieee30/Line 1-3-2 ==
  Line{,1..4} (5 alike) : powerlib/Elements/Three-Phase PI Section Line  LConnTagsString=a|b|c  RConnTagsString=A|B|C  Frequency=60  Resistances=[rt ro] /100  Inductances=[ lt lo] /100  Capacitances=[ct co]/100  Length=20
      settings: SourceProductName=Simscape Power Systems
  A : PMIOPort  Port=1  Side=Left
  B : PMIOPort  Port=2  Side=Left
  C : PMIOPort  Port=3  Side=Left
  a : PMIOPort  Port=4  Side=Right
  b : PMIOPort  Port=5  Side=Right
  c : PMIOPort  Port=6  Side=Right
  connections:
  Line3/RConn3 -- Line4/LConn3
  Line/RConn3 -- Line1/LConn3
  Line2/RConn3 -- Line3/LConn3
  Line2/RConn1 -- Line3/LConn1
  Line1/RConn3 -- Line2/LConn3
  Line/RConn2 -- Line1/LConn2
  Line2/RConn2 -- Line3/LConn2
  Line1/RConn1 -- Line2/LConn1
  Line3/RConn1 -- Line4/LConn1
  Line3/RConn2 -- Line4/LConn2
  Line1/RConn2 -- Line2/LConn2
  Line/RConn1 -- Line1/LConn1
  C/RConn1 -- Line/LConn3
  Line/LConn1 -- A/RConn1
  c/RConn1 -- Line4/RConn3
  a/RConn1 -- Line4/RConn1
  B/RConn1 -- Line/LConn2
  b/RConn1 -- Line4/RConn2

== system ieee30/Line 10-17-1 ==
  Line{,1..4} (5 alike) : powerlib/Elements/Three-Phase PI Section Line  LConnTagsString=a|b|c  RConnTagsString=A|B|C  Frequency=60  Resistances=[rt ro] /100  Inductances=[ lt lo] /100  Capacitances=[ct co]/100  Length=20
      settings: SourceProductName=Simscape Power Systems
  A : PMIOPort  Port=1  Side=Left
  B : PMIOPort  Port=2  Side=Left
  C : PMIOPort  Port=3  Side=Left
  a : PMIOPort  Port=4  Side=Right
  b : PMIOPort  Port=5  Side=Right
  c : PMIOPort  Port=6  Side=Right
  connections:
  Line3/RConn3 -- Line4/LConn3
  Line/RConn3 -- Line1/LConn3
  Line2/RConn3 -- Line3/LConn3
  Line2/RConn1 -- Line3/LConn1
  Line1/RConn3 -- Line2/LConn3
  Line/RConn2 -- Line1/LConn2
  Line2/RConn2 -- Line3/LConn2
  Line1/RConn1 -- Line2/LConn1
  Line3/RConn1 -- Line4/LConn1
  Line3/RConn2 -- Line4/LConn2
  Line1/RConn2 -- Line2/LConn2
  Line/RConn1 -- Line1/LConn1
  C/RConn1 -- Line/LConn3
  Line/LConn1 -- A/RConn1
  c/RConn1 -- Line4/RConn3
  a/RConn1 -- Line4/RConn1
  B/RConn1 -- Line/LConn2
  b/RConn1 -- Line4/RConn2

== system ieee30/Line 10-17-2 ==
  Line{,1..4} (5 alike) : powerlib/Elements/Three-Phase PI Section Line  LConnTagsString=a|b|c  RConnTagsString=A|B|C  Frequency=60  Resistances=[rt ro] /100  Inductances=[ lt lo] /100  Capacitances=[ct co]/100  Length=20
      settings: SourceProductName=Simscape Power Systems
  A : PMIOPort  Port=1  Side=Left
  B : PMIOPort  Port=2  Side=Left
  C : PMIOPort  Port=3  Side=Left
  a : PMIOPort  Port=4  Side=Right
  b : PMIOPort  Port=5  Side=Right
  c : PMIOPort  Port=6  Side=Right
  connections:
  Line3/RConn3 -- Line4/LConn3
  Line/RConn3 -- Line1/LConn3
  Line2/RConn3 -- Line3/LConn3
  Line2/RConn1 -- Line3/LConn1
  Line1/RConn3 -- Line2/LConn3
  Line/RConn2 -- Line1/LConn2
  Line2/RConn2 -- Line3/LConn2
  Line1/RConn1 -- Line2/LConn1
  Line3/RConn1 -- Line4/LConn1
  Line3/RConn2 -- Line4/LConn2
  Line1/RConn2 -- Line2/LConn2
  Line/RConn1 -- Line1/LConn1
  C/RConn1 -- Line/LConn3
  Line/LConn1 -- A/RConn1
  c/RConn1 -- Line4/RConn3
  a/RConn1 -- Line4/RConn1
  B/RConn1 -- Line/LConn2
  b/RConn1 -- Line4/RConn2

== system ieee30/Line 10-20-1 ==
  Line{,1..4} (5 alike) : powerlib/Elements/Three-Phase PI Section Line  LConnTagsString=a|b|c  RConnTagsString=A|B|C  Frequency=60  Resistances=[rt ro] /100  Inductances=[ lt lo] /100  Capacitances=[ct co]/100  Length=20
      settings: SourceProductName=Simscape Power Systems
  A : PMIOPort  Port=1  Side=Left
  B : PMIOPort  Port=2  Side=Left
  C : PMIOPort  Port=3  Side=Left
  a : PMIOPort  Port=4  Side=Right
  b : PMIOPort  Port=5  Side=Right
  c : PMIOPort  Port=6  Side=Right
  connections:
  Line3/RConn3 -- Line4/LConn3
  Line/RConn3 -- Line1/LConn3
  Line2/RConn3 -- Line3/LConn3
  Line2/RConn1 -- Line3/LConn1
  Line1/RConn3 -- Line2/LConn3
  Line/RConn2 -- Line1/LConn2
  Line2/RConn2 -- Line3/LConn2
  Line1/RConn1 -- Line2/LConn1
  Line3/RConn1 -- Line4/LConn1
  Line3/RConn2 -- Line4/LConn2
  Line1/RConn2 -- Line2/LConn2
  Line/RConn1 -- Line1/LConn1
  C/RConn1 -- Line/LConn3
  Line/LConn1 -- A/RConn1
  c/RConn1 -- Line4/RConn3
  a/RConn1 -- Line4/RConn1
  B/RConn1 -- Line/LConn2
  b/RConn1 -- Line4/RConn2

== system ieee30/Line 10-20-2 ==
  Line{,1..4} (5 alike) : powerlib/Elements/Three-Phase PI Section Line  LConnTagsString=a|b|c  RConnTagsString=A|B|C  Frequency=60  Resistances=[rt ro] /100  Inductances=[ lt lo] /100  Capacitances=[ct co]/100  Length=20
      settings: SourceProductName=Simscape Power Systems
  A : PMIOPort  Port=1  Side=Left
  B : PMIOPort  Port=2  Side=Left
  C : PMIOPort  Port=3  Side=Left
  a : PMIOPort  Port=4  Side=Right
  b : PMIOPort  Port=5  Side=Right
  c : PMIOPort  Port=6  Side=Right
  connections:
  Line3/RConn3 -- Line4/LConn3
  Line/RConn3 -- Line1/LConn3
  Line2/RConn3 -- Line3/LConn3
  Line2/RConn1 -- Line3/LConn1
  Line1/RConn3 -- Line2/LConn3
  Line/RConn2 -- Line1/LConn2
  Line2/RConn2 -- Line3/LConn2
  Line1/RConn1 -- Line2/LConn1
  Line3/RConn1 -- Line4/LConn1
  Line3/RConn2 -- Line4/LConn2
  Line1/RConn2 -- Line2/LConn2
  Line/RConn1 -- Line1/LConn1
  C/RConn1 -- Line/LConn3
  Line/LConn1 -- A/RConn1
  c/RConn1 -- Line4/RConn3
  a/RConn1 -- Line4/RConn1
  B/RConn1 -- Line/LConn2
  b/RConn1 -- Line4/RConn2

== system ieee30/Line 10-21-1 ==
  Line{,1..4} (5 alike) : powerlib/Elements/Three-Phase PI Section Line  LConnTagsString=a|b|c  RConnTagsString=A|B|C  Frequency=60  Resistances=[rt ro] /100  Inductances=[ lt lo] /100  Capacitances=[ct co]/100  Length=20
      settings: SourceProductName=Simscape Power Systems
  A : PMIOPort  Port=1  Side=Left
  B : PMIOPort  Port=2  Side=Left
  C : PMIOPort  Port=3  Side=Left
  a : PMIOPort  Port=4  Side=Right
  b : PMIOPort  Port=5  Side=Right
  c : PMIOPort  Port=6  Side=Right
  connections:
  Line3/RConn3 -- Line4/LConn3
  Line/RConn3 -- Line1/LConn3
  Line2/RConn3 -- Line3/LConn3
  Line2/RConn1 -- Line3/LConn1
  Line1/RConn3 -- Line2/LConn3
  Line/RConn2 -- Line1/LConn2
  Line2/RConn2 -- Line3/LConn2
  Line1/RConn1 -- Line2/LConn1
  Line3/RConn1 -- Line4/LConn1
  Line3/RConn2 -- Line4/LConn2
  Line1/RConn2 -- Line2/LConn2
  Line/RConn1 -- Line1/LConn1
  C/RConn1 -- Line/LConn3
  Line/LConn1 -- A/RConn1
  c/RConn1 -- Line4/RConn3
  a/RConn1 -- Line4/RConn1
  B/RConn1 -- Line/LConn2
  b/RConn1 -- Line4/RConn2

== system ieee30/Line 10-21-2 ==
  Line{,1..4} (5 alike) : powerlib/Elements/Three-Phase PI Section Line  LConnTagsString=a|b|c  RConnTagsString=A|B|C  Frequency=60  Resistances=[rt ro] /100  Inductances=[ lt lo] /100  Capacitances=[ct co]/100  Length=20
      settings: SourceProductName=Simscape Power Systems
  A : PMIOPort  Port=1  Side=Left
  B : PMIOPort  Port=2  Side=Left
  C : PMIOPort  Port=3  Side=Left
  a : PMIOPort  Port=4  Side=Right
  b : PMIOPort  Port=5  Side=Right
  c : PMIOPort  Port=6  Side=Right
  connections:
  Line3/RConn3 -- Line4/LConn3
  Line/RConn3 -- Line1/LConn3
  Line2/RConn3 -- Line3/LConn3
  Line2/RConn1 -- Line3/LConn1
  Line1/RConn3 -- Line2/LConn3
  Line/RConn2 -- Line1/LConn2
  Line2/RConn2 -- Line3/LConn2
  Line1/RConn1 -- Line2/LConn1
  Line3/RConn1 -- Line4/LConn1
  Line3/RConn2 -- Line4/LConn2
  Line1/RConn2 -- Line2/LConn2
  Line/RConn1 -- Line1/LConn1
  C/RConn1 -- Line/LConn3
  Line/LConn1 -- A/RConn1
  c/RConn1 -- Line4/RConn3
  a/RConn1 -- Line4/RConn1
  B/RConn1 -- Line/LConn2
  b/RConn1 -- Line4/RConn2

== system ieee30/Line 10-22-1 ==
  Line{,1..4} (5 alike) : powerlib/Elements/Three-Phase PI Section Line  LConnTagsString=a|b|c  RConnTagsString=A|B|C  Frequency=60  Resistances=[rt ro] /100  Inductances=[ lt lo] /100  Capacitances=[ct co]/100  Length=20
      settings: SourceProductName=Simscape Power Systems
  A : PMIOPort  Port=1  Side=Left
  B : PMIOPort  Port=2  Side=Left
  C : PMIOPort  Port=3  Side=Left
  a : PMIOPort  Port=4  Side=Right
  b : PMIOPort  Port=5  Side=Right
  c : PMIOPort  Port=6  Side=Right
  connections:
  Line3/RConn3 -- Line4/LConn3
  Line/RConn3 -- Line1/LConn3
  Line2/RConn3 -- Line3/LConn3
  Line2/RConn1 -- Line3/LConn1
  Line1/RConn3 -- Line2/LConn3
  Line/RConn2 -- Line1/LConn2
  Line2/RConn2 -- Line3/LConn2
  Line1/RConn1 -- Line2/LConn1
  Line3/RConn1 -- Line4/LConn1
  Line3/RConn2 -- Line4/LConn2
  Line1/RConn2 -- Line2/LConn2
  Line/RConn1 -- Line1/LConn1
  C/RConn1 -- Line/LConn3
  Line/LConn1 -- A/RConn1
  c/RConn1 -- Line4/RConn3
  a/RConn1 -- Line4/RConn1
  B/RConn1 -- Line/LConn2
  b/RConn1 -- Line4/RConn2

== system ieee30/Line 10-22-2 ==
  Line{,1..4} (5 alike) : powerlib/Elements/Three-Phase PI Section Line  LConnTagsString=a|b|c  RConnTagsString=A|B|C  Frequency=60  Resistances=[rt ro] /100  Inductances=[ lt lo] /100  Capacitances=[ct co]/100  Length=20
      settings: SourceProductName=Simscape Power Systems
  A : PMIOPort  Port=1  Side=Left
  B : PMIOPort  Port=2  Side=Left
  C : PMIOPort  Port=3  Side=Left
  a : PMIOPort  Port=4  Side=Right
  b : PMIOPort  Port=5  Side=Right
  c : PMIOPort  Port=6  Side=Right
  connections:
  Line3/RConn3 -- Line4/LConn3
  Line/RConn3 -- Line1/LConn3
  Line2/RConn3 -- Line3/LConn3
  Line2/RConn1 -- Line3/LConn1
  Line1/RConn3 -- Line2/LConn3
  Line/RConn2 -- Line1/LConn2
  Line2/RConn2 -- Line3/LConn2
  Line1/RConn1 -- Line2/LConn1
  Line3/RConn1 -- Line4/LConn1
  Line3/RConn2 -- Line4/LConn2
  Line1/RConn2 -- Line2/LConn2
  Line/RConn1 -- Line1/LConn1
  C/RConn1 -- Line/LConn3
  Line/LConn1 -- A/RConn1
  c/RConn1 -- Line4/RConn3
  a/RConn1 -- Line4/RConn1
  B/RConn1 -- Line/LConn2
  b/RConn1 -- Line4/RConn2

== system ieee30/Line 12-14-1 ==
  Line{,1..4} (5 alike) : powerlib/Elements/Three-Phase PI Section Line  LConnTagsString=a|b|c  RConnTagsString=A|B|C  Frequency=60  Resistances=[rt ro] /100  Inductances=[ lt lo] /100  Capacitances=[ct co]/100  Length=20
      settings: SourceProductName=Simscape Power Systems
  A : PMIOPort  Port=1  Side=Left
  B : PMIOPort  Port=2  Side=Left
  C : PMIOPort  Port=3  Side=Left
  a : PMIOPort  Port=4  Side=Right
  b : PMIOPort  Port=5  Side=Right
  c : PMIOPort  Port=6  Side=Right
  connections:
  Line3/RConn3 -- Line4/LConn3
  Line/RConn3 -- Line1/LConn3
  Line2/RConn3 -- Line3/LConn3
  Line2/RConn1 -- Line3/LConn1
  Line1/RConn3 -- Line2/LConn3
  Line/RConn2 -- Line1/LConn2
  Line2/RConn2 -- Line3/LConn2
  Line1/RConn1 -- Line2/LConn1
  Line3/RConn1 -- Line4/LConn1
  Line3/RConn2 -- Line4/LConn2
  Line1/RConn2 -- Line2/LConn2
  Line/RConn1 -- Line1/LConn1
  C/RConn1 -- Line/LConn3
  Line/LConn1 -- A/RConn1
  c/RConn1 -- Line4/RConn3
  a/RConn1 -- Line4/RConn1
  B/RConn1 -- Line/LConn2
  b/RConn1 -- Line4/RConn2

== system ieee30/Line 12-14-2 ==
  Line{,1..4} (5 alike) : powerlib/Elements/Three-Phase PI Section Line  LConnTagsString=a|b|c  RConnTagsString=A|B|C  Frequency=60  Resistances=[rt ro] /100  Inductances=[ lt lo] /100  Capacitances=[ct co]/100  Length=20
      settings: SourceProductName=Simscape Power Systems
  A : PMIOPort  Port=1  Side=Left
  B : PMIOPort  Port=2  Side=Left
  C : PMIOPort  Port=3  Side=Left
  a : PMIOPort  Port=4  Side=Right
  b : PMIOPort  Port=5  Side=Right
  c : PMIOPort  Port=6  Side=Right
  connections:
  Line3/RConn3 -- Line4/LConn3
  Line/RConn3 -- Line1/LConn3
  Line2/RConn3 -- Line3/LConn3
  Line2/RConn1 -- Line3/LConn1
  Line1/RConn3 -- Line2/LConn3
  Line/RConn2 -- Line1/LConn2
  Line2/RConn2 -- Line3/LConn2
  Line1/RConn1 -- Line2/LConn1
  Line3/RConn1 -- Line4/LConn1
  Line3/RConn2 -- Line4/LConn2
  Line1/RConn2 -- Line2/LConn2
  Line/RConn1 -- Line1/LConn1
  C/RConn1 -- Line/LConn3
  Line/LConn1 -- A/RConn1
  c/RConn1 -- Line4/RConn3
  a/RConn1 -- Line4/RConn1
  B/RConn1 -- Line/LConn2
  b/RConn1 -- Line4/RConn2

== system ieee30/Line 12-15-1 ==
  Line{,1..4} (5 alike) : powerlib/Elements/Three-Phase PI Section Line  LConnTagsString=a|b|c  RConnTagsString=A|B|C  Frequency=60  Resistances=[rt ro] /100  Inductances=[ lt lo] /100  Capacitances=[ct co]/100  Length=20
      settings: SourceProductName=Simscape Power Systems
  A : PMIOPort  Port=1  Side=Left
  B : PMIOPort  Port=2  Side=Left
  C : PMIOPort  Port=3  Side=Left
  a : PMIOPort  Port=4  Side=Right
  b : PMIOPort  Port=5  Side=Right
  c : PMIOPort  Port=6  Side=Right
  connections:
  Line3/RConn3 -- Line4/LConn3
  Line/RConn3 -- Line1/LConn3
  Line2/RConn3 -- Line3/LConn3
  Line2/RConn1 -- Line3/LConn1
  Line1/RConn3 -- Line2/LConn3
  Line/RConn2 -- Line1/LConn2
  Line2/RConn2 -- Line3/LConn2
  Line1/RConn1 -- Line2/LConn1
  Line3/RConn1 -- Line4/LConn1
  Line3/RConn2 -- Line4/LConn2
  Line1/RConn2 -- Line2/LConn2
  Line/RConn1 -- Line1/LConn1
  C/RConn1 -- Line/LConn3
  Line/LConn1 -- A/RConn1
  c/RConn1 -- Line4/RConn3
  a/RConn1 -- Line4/RConn1
  B/RConn1 -- Line/LConn2
  b/RConn1 -- Line4/RConn2

== system ieee30/Line 12-15-2 ==
  Line{,1..4} (5 alike) : powerlib/Elements/Three-Phase PI Section Line  LConnTagsString=a|b|c  RConnTagsString=A|B|C  Frequency=60  Resistances=[rt ro] /100  Inductances=[ lt lo] /100  Capacitances=[ct co]/100  Length=20
      settings: SourceProductName=Simscape Power Systems
  A : PMIOPort  Port=1  Side=Left
  B : PMIOPort  Port=2  Side=Left
  C : PMIOPort  Port=3  Side=Left
  a : PMIOPort  Port=4  Side=Right
  b : PMIOPort  Port=5  Side=Right
  c : PMIOPort  Port=6  Side=Right
  connections:
  Line3/RConn3 -- Line4/LConn3
  Line/RConn3 -- Line1/LConn3
  Line2/RConn3 -- Line3/LConn3
  Line2/RConn1 -- Line3/LConn1
  Line1/RConn3 -- Line2/LConn3
  Line/RConn2 -- Line1/LConn2
  Line2/RConn2 -- Line3/LConn2
  Line1/RConn1 -- Line2/LConn1
  Line3/RConn1 -- Line4/LConn1
  Line3/RConn2 -- Line4/LConn2
  Line1/RConn2 -- Line2/LConn2
  Line/RConn1 -- Line1/LConn1
  C/RConn1 -- Line/LConn3
  Line/LConn1 -- A/RConn1
  c/RConn1 -- Line4/RConn3
  a/RConn1 -- Line4/RConn1
  B/RConn1 -- Line/LConn2
  b/RConn1 -- Line4/RConn2

== system ieee30/Line 12-16-1 ==
  Line{,1..4} (5 alike) : powerlib/Elements/Three-Phase PI Section Line  LConnTagsString=a|b|c  RConnTagsString=A|B|C  Frequency=60  Resistances=[rt ro] /100  Inductances=[ lt lo] /100  Capacitances=[ct co]/100  Length=20
      settings: SourceProductName=Simscape Power Systems
  A : PMIOPort  Port=1  Side=Left
  B : PMIOPort  Port=2  Side=Left
  C : PMIOPort  Port=3  Side=Left
  a : PMIOPort  Port=4  Side=Right
  b : PMIOPort  Port=5  Side=Right
  c : PMIOPort  Port=6  Side=Right
  connections:
  Line3/RConn3 -- Line4/LConn3
  Line/RConn3 -- Line1/LConn3
  Line2/RConn3 -- Line3/LConn3
  Line2/RConn1 -- Line3/LConn1
  Line1/RConn3 -- Line2/LConn3
  Line/RConn2 -- Line1/LConn2
  Line2/RConn2 -- Line3/LConn2
  Line1/RConn1 -- Line2/LConn1
  Line3/RConn1 -- Line4/LConn1
  Line3/RConn2 -- Line4/LConn2
  Line1/RConn2 -- Line2/LConn2
  Line/RConn1 -- Line1/LConn1
  C/RConn1 -- Line/LConn3
  Line/LConn1 -- A/RConn1
  c/RConn1 -- Line4/RConn3
  a/RConn1 -- Line4/RConn1
  B/RConn1 -- Line/LConn2
  b/RConn1 -- Line4/RConn2

== system ieee30/Line 12-16-2 ==
  Line{,1..4} (5 alike) : powerlib/Elements/Three-Phase PI Section Line  LConnTagsString=a|b|c  RConnTagsString=A|B|C  Frequency=60  Resistances=[rt ro] /100  Inductances=[ lt lo] /100  Capacitances=[ct co]/100  Length=20
      settings: SourceProductName=Simscape Power Systems
  A : PMIOPort  Port=1  Side=Left
  B : PMIOPort  Port=2  Side=Left
  C : PMIOPort  Port=3  Side=Left
  a : PMIOPort  Port=4  Side=Right
  b : PMIOPort  Port=5  Side=Right
  c : PMIOPort  Port=6  Side=Right
  connections:
  Line3/RConn3 -- Line4/LConn3
  Line/RConn3 -- Line1/LConn3
  Line2/RConn3 -- Line3/LConn3
  Line2/RConn1 -- Line3/LConn1
  Line1/RConn3 -- Line2/LConn3
  Line/RConn2 -- Line1/LConn2
  Line2/RConn2 -- Line3/LConn2
  Line1/RConn1 -- Line2/LConn1
  Line3/RConn1 -- Line4/LConn1
  Line3/RConn2 -- Line4/LConn2
  Line1/RConn2 -- Line2/LConn2
  Line/RConn1 -- Line1/LConn1
  C/RConn1 -- Line/LConn3
  Line/LConn1 -- A/RConn1
  c/RConn1 -- Line4/RConn3
  a/RConn1 -- Line4/RConn1
  B/RConn1 -- Line/LConn2
  b/RConn1 -- Line4/RConn2

== system ieee30/Line 14-15-1 ==
  Line{,1..4} (5 alike) : powerlib/Elements/Three-Phase PI Section Line  LConnTagsString=a|b|c  RConnTagsString=A|B|C  Frequency=60  Resistances=[rt ro] /100  Inductances=[ lt lo] /100  Capacitances=[ct co]/100  Length=20
      settings: SourceProductName=Simscape Power Systems
  A : PMIOPort  Port=1  Side=Left
  B : PMIOPort  Port=2  Side=Left
  C : PMIOPort  Port=3  Side=Left
  a : PMIOPort  Port=4  Side=Right
  b : PMIOPort  Port=5  Side=Right
  c : PMIOPort  Port=6  Side=Right
  connections:
  Line3/RConn3 -- Line4/LConn3
  Line/RConn3 -- Line1/LConn3
  Line2/RConn3 -- Line3/LConn3
  Line2/RConn1 -- Line3/LConn1
  Line1/RConn3 -- Line2/LConn3
  Line/RConn2 -- Line1/LConn2
  Line2/RConn2 -- Line3/LConn2
  Line1/RConn1 -- Line2/LConn1
  Line3/RConn1 -- Line4/LConn1
  Line3/RConn2 -- Line4/LConn2
  Line1/RConn2 -- Line2/LConn2
  Line/RConn1 -- Line1/LConn1
  C/RConn1 -- Line/LConn3
  Line/LConn1 -- A/RConn1
  c/RConn1 -- Line4/RConn3
  a/RConn1 -- Line4/RConn1
  B/RConn1 -- Line/LConn2
  b/RConn1 -- Line4/RConn2

== system ieee30/Line 14-15-2 ==
  Line{,1..4} (5 alike) : powerlib/Elements/Three-Phase PI Section Line  LConnTagsString=a|b|c  RConnTagsString=A|B|C  Frequency=60  Resistances=[rt ro] /100  Inductances=[ lt lo] /100  Capacitances=[ct co]/100  Length=20
      settings: SourceProductName=Simscape Power Systems
  A : PMIOPort  Port=1  Side=Left
  B : PMIOPort  Port=2  Side=Left
  C : PMIOPort  Port=3  Side=Left
  a : PMIOPort  Port=4  Side=Right
  b : PMIOPort  Port=5  Side=Right
  c : PMIOPort  Port=6  Side=Right
  connections:
  Line3/RConn3 -- Line4/LConn3
  Line/RConn3 -- Line1/LConn3
  Line2/RConn3 -- Line3/LConn3
  Line2/RConn1 -- Line3/LConn1
  Line1/RConn3 -- Line2/LConn3
  Line/RConn2 -- Line1/LConn2
  Line2/RConn2 -- Line3/LConn2
  Line1/RConn1 -- Line2/LConn1
  Line3/RConn1 -- Line4/LConn1
  Line3/RConn2 -- Line4/LConn2
  Line1/RConn2 -- Line2/LConn2
  Line/RConn1 -- Line1/LConn1
  C/RConn1 -- Line/LConn3
  Line/LConn1 -- A/RConn1
  c/RConn1 -- Line4/RConn3
  a/RConn1 -- Line4/RConn1
  B/RConn1 -- Line/LConn2
  b/RConn1 -- Line4/RConn2

== system ieee30/Line 15-18-1 ==
  Line{,1..4} (5 alike) : powerlib/Elements/Three-Phase PI Section Line  LConnTagsString=a|b|c  RConnTagsString=A|B|C  Frequency=60  Resistances=[rt ro] /100  Inductances=[ lt lo] /100  Capacitances=[ct co]/100  Length=20
      settings: SourceProductName=Simscape Power Systems
  A : PMIOPort  Port=1  Side=Left
  B : PMIOPort  Port=2  Side=Left
  C : PMIOPort  Port=3  Side=Left
  a : PMIOPort  Port=4  Side=Right
  b : PMIOPort  Port=5  Side=Right
  c : PMIOPort  Port=6  Side=Right
  connections:
  Line3/RConn3 -- Line4/LConn3
  Line/RConn3 -- Line1/LConn3
  Line2/RConn3 -- Line3/LConn3
  Line2/RConn1 -- Line3/LConn1
  Line1/RConn3 -- Line2/LConn3
  Line/RConn2 -- Line1/LConn2
  Line2/RConn2 -- Line3/LConn2
  Line1/RConn1 -- Line2/LConn1
  Line3/RConn1 -- Line4/LConn1
  Line3/RConn2 -- Line4/LConn2
  Line1/RConn2 -- Line2/LConn2
  Line/RConn1 -- Line1/LConn1
  C/RConn1 -- Line/LConn3
  Line/LConn1 -- A/RConn1
  c/RConn1 -- Line4/RConn3
  a/RConn1 -- Line4/RConn1
  B/RConn1 -- Line/LConn2
  b/RConn1 -- Line4/RConn2

== system ieee30/Line 15-18-2 ==
  Line{,1..4} (5 alike) : powerlib/Elements/Three-Phase PI Section Line  LConnTagsString=a|b|c  RConnTagsString=A|B|C  Frequency=60  Resistances=[rt ro] /100  Inductances=[ lt lo] /100  Capacitances=[ct co]/100  Length=20
      settings: SourceProductName=Simscape Power Systems
  A : PMIOPort  Port=1  Side=Left
  B : PMIOPort  Port=2  Side=Left
  C : PMIOPort  Port=3  Side=Left
  a : PMIOPort  Port=4  Side=Right
  b : PMIOPort  Port=5  Side=Right
  c : PMIOPort  Port=6  Side=Right
  connections:
  Line3/RConn3 -- Line4/LConn3
  Line/RConn3 -- Line1/LConn3
  Line2/RConn3 -- Line3/LConn3
  Line2/RConn1 -- Line3/LConn1
  Line1/RConn3 -- Line2/LConn3
  Line/RConn2 -- Line1/LConn2
  Line2/RConn2 -- Line3/LConn2
  Line1/RConn1 -- Line2/LConn1
  Line3/RConn1 -- Line4/LConn1
  Line3/RConn2 -- Line4/LConn2
  Line1/RConn2 -- Line2/LConn2
  Line/RConn1 -- Line1/LConn1
  C/RConn1 -- Line/LConn3
  Line/LConn1 -- A/RConn1
  c/RConn1 -- Line4/RConn3
  a/RConn1 -- Line4/RConn1
  B/RConn1 -- Line/LConn2
  b/RConn1 -- Line4/RConn2

== system ieee30/Line 15-23-1 ==
  Line{,1..4} (5 alike) : powerlib/Elements/Three-Phase PI Section Line  LConnTagsString=a|b|c  RConnTagsString=A|B|C  Frequency=60  Resistances=[rt ro] /100  Inductances=[ lt lo] /100  Capacitances=[ct co]/100  Length=20
      settings: SourceProductName=Simscape Power Systems
  A : PMIOPort  Port=1  Side=Left
  B : PMIOPort  Port=2  Side=Left
  C : PMIOPort  Port=3  Side=Left
  a : PMIOPort  Port=4  Side=Right
  b : PMIOPort  Port=5  Side=Right
  c : PMIOPort  Port=6  Side=Right
  connections:
  Line3/RConn3 -- Line4/LConn3
  Line/RConn3 -- Line1/LConn3
  Line2/RConn3 -- Line3/LConn3
  Line2/RConn1 -- Line3/LConn1
  Line1/RConn3 -- Line2/LConn3
  Line/RConn2 -- Line1/LConn2
  Line2/RConn2 -- Line3/LConn2
  Line1/RConn1 -- Line2/LConn1
  Line3/RConn1 -- Line4/LConn1
  Line3/RConn2 -- Line4/LConn2
  Line1/RConn2 -- Line2/LConn2
  Line/RConn1 -- Line1/LConn1
  C/RConn1 -- Line/LConn3
  Line/LConn1 -- A/RConn1
  c/RConn1 -- Line4/RConn3
  a/RConn1 -- Line4/RConn1
  B/RConn1 -- Line/LConn2
  b/RConn1 -- Line4/RConn2

== system ieee30/Line 15-23-2 ==
  Line{,1..4} (5 alike) : powerlib/Elements/Three-Phase PI Section Line  LConnTagsString=a|b|c  RConnTagsString=A|B|C  Frequency=60  Resistances=[rt ro] /100  Inductances=[ lt lo] /100  Capacitances=[ct co]/100  Length=20
      settings: SourceProductName=Simscape Power Systems
  A : PMIOPort  Port=1  Side=Left
  B : PMIOPort  Port=2  Side=Left
  C : PMIOPort  Port=3  Side=Left
  a : PMIOPort  Port=4  Side=Right
  b : PMIOPort  Port=5  Side=Right
  c : PMIOPort  Port=6  Side=Right
  connections:
  Line3/RConn3 -- Line4/LConn3
  Line/RConn3 -- Line1/LConn3
  Line2/RConn3 -- Line3/LConn3
  Line2/RConn1 -- Line3/LConn1
  Line1/RConn3 -- Line2/LConn3
  Line/RConn2 -- Line1/LConn2
  Line2/RConn2 -- Line3/LConn2
  Line1/RConn1 -- Line2/LConn1
  Line3/RConn1 -- Line4/LConn1
  Line3/RConn2 -- Line4/LConn2
  Line1/RConn2 -- Line2/LConn2
  Line/RConn1 -- Line1/LConn1
  C/RConn1 -- Line/LConn3
  Line/LConn1 -- A/RConn1
  c/RConn1 -- Line4/RConn3
  a/RConn1 -- Line4/RConn1
  B/RConn1 -- Line/LConn2
  b/RConn1 -- Line4/RConn2

== system ieee30/Line 16-17-1 ==
  Line{,1..4} (5 alike) : powerlib/Elements/Three-Phase PI Section Line  LConnTagsString=a|b|c  RConnTagsString=A|B|C  Frequency=60  Resistances=[rt ro] /100  Inductances=[ lt lo] /100  Capacitances=[ct co]/100  Length=20
      settings: SourceProductName=Simscape Power Systems
  A : PMIOPort  Port=1  Side=Left
  B : PMIOPort  Port=2  Side=Left
  C : PMIOPort  Port=3  Side=Left
  a : PMIOPort  Port=4  Side=Right
  b : PMIOPort  Port=5  Side=Right
  c : PMIOPort  Port=6  Side=Right
  connections:
  Line3/RConn3 -- Line4/LConn3
  Line/RConn3 -- Line1/LConn3
  Line2/RConn3 -- Line3/LConn3
  Line2/RConn1 -- Line3/LConn1
  Line1/RConn3 -- Line2/LConn3
  Line/RConn2 -- Line1/LConn2
  Line2/RConn2 -- Line3/LConn2
  Line1/RConn1 -- Line2/LConn1
  Line3/RConn1 -- Line4/LConn1
  Line3/RConn2 -- Line4/LConn2
  Line1/RConn2 -- Line2/LConn2
  Line/RConn1 -- Line1/LConn1
  C/RConn1 -- Line/LConn3
  Line/LConn1 -- A/RConn1
  c/RConn1 -- Line4/RConn3
  a/RConn1 -- Line4/RConn1
  B/RConn1 -- Line/LConn2
  b/RConn1 -- Line4/RConn2
